simulink model "Model"  (R2021b)
settings: Solver=FixedStepAuto  StartTime=0.0  StopTime=T  FixedStep=0.1  RelTol=1e-3
values from neighbouring files (symbols this model uses):
  A = zeros(length(w_0))    [Model_script.m]
  a = R_E + 550    [Model_script.m]    (also in Orbit_Model.m)
  A0 = eye(3)    [Model_script.m]
  actuators_matrix = [1 0 0; 0 1 0; 0 0 1]    [Model_script.m]
  alpha = deg2rad(11.5)    [Model_script.m]
  Area_mb = diag([A1 A2 A3 A4 A5 A6])    [Model_script.m]
  Area_sp = diag([A7 A8 A9 A10])    [Model_script.m]
  around_boresight = deg2rad(dms2degrees([0,0,around_boresight]))    [Model_script.m]
  B = diag([1/Ix, 1/Iy, 1/Iz])    [Model_script.m]
  cross_boresight = deg2rad(dms2degrees([0,0,cross_boresight]))    [Model_script.m]
  e = 0.0001824    [Model_script.m]    (also in Orbit_Model.m)
  epsilon = deg2rad(23.45)    [Model_script.m]
  H0 = ( g1_0^2 + g1_1^2 + h1_1^2 )^(1/2)    (= 3.0115258674e-05)    [Model_script.m]
  h_N_target = [0; 0; I(3,3)*n]    [Model_script.m]
  I = I_mb + I_depl    [Model_script.m]
  i = deg2rad(53.0545)    [Model_script.m]    (also in Orbit_Model.m)
  I_inv = inv(I)    [Model_script.m]
  i_matrix = [1 0 0; 0 cos(i) sin(i); 0 -sin(i) cos(i)]    [Model_script.m]
  Kb = 1e10    (= 10000000000)    [Model_script.m]
  Kd = 5*1e-4*ones(length(w_0),1)    [Model_script.m]
  Kp = 5*1e-3*ones(length(w_0),1)    [Model_script.m]
  m = [0.01; 0.05; 0.01]    [Model_script.m]
  m_N_unit = zeros(size(m_N,1),size(m_N,2))    [Model_script.m]
  mu_E = astroConstants(13)    [Model_script.m]    (also in Orbit_Model.m)
  n = sqrt(mu_E/(a^3))    [Model_script.m]    (also in Orbit_Model.m)
  n4 = -n1    [Model_script.m]
  N_b_mb = [n1'; n2'; n3'; n4'; n5'; n6']    [Model_script.m]
  N_b_sp = [n7'; n8'; n9'; n10']    [Model_script.m]
  n_sun = 2*pi/T_sun    (= 1.99238499086e-07)    [Model_script.m]
  P = Fe/c    (= 4.52666666667e-06)    [Model_script.m]
  Q = zeros(length(w_0))    [Model_script.m]
  R = zeros(length(w_0))    [Model_script.m]
  R_E = astroConstants(23)    [Model_script.m]    (also in Orbit_Model.m)
  r_mb = [base/2 0 0; 0 base/2 0; 0 0 height/2; -base/2 0 0; 0 -base/2 0; 0 0 -height/2]    [Model_script.m]
  r_sp = [0 length_p1/2+base/2 0; 0 length_p1/2+base/2 0; 0 -length_p2/2-base/2 0; 0 -length_p2/2-base/2 0]    [Model_script.m]
  rho_s_mb = 0.3    [Model_script.m]
  rho_s_sp = 0    [Model_script.m]
  Rs = astroConstants(2)    [Model_script.m]
  star_sensor_tolerance = deg2rad(star_sensor_tolerance)    [Model_script.m]
  theta0 = deg2rad(0)    [Model_script.m]    (also in Orbit_Model.m)
  unit = [1 0 0]'    [Model_script.m]
  v1 = [0 1 -1]'    [Model_script.m]
  v2 = [-1 0 1]'    [Model_script.m]
  v3 = [1 -1 0]'    [Model_script.m]
  w_0 = [wx_0 wy_0 wz_0]'    [Model_script.m]
  w_E = deg2rad(15.04)/3600    [Model_script.m]    (also in Orbit_Model.m = deg2rad(15.04/3600))
  w_target = [0; 0; n]    [Model_script.m]
  weight = 1/6    (= 0.166666666667)    [Model_script.m]
  wy_0 = 0.7    [Model_script.m]
undefined symbols (not defined in the file or in its folder): phi0, psi0, q0
libraries: matrix_library x15, vrlib x12, dspmtrx3 x3, sharedutil x2
(part 1 of 2)
settings Model: Creator=sferl  LastModifiedBy=samuz

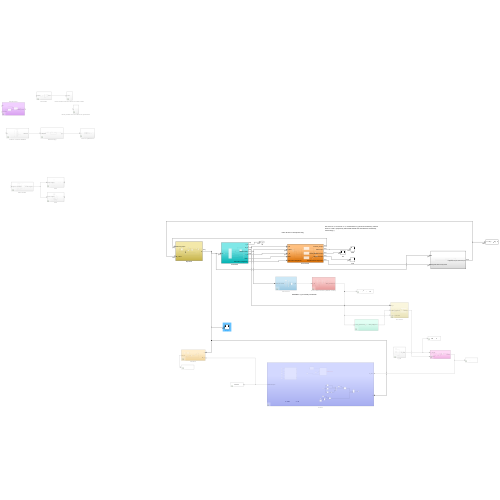
[thumbnail: Simulink's stored preview of the top-level diagram]
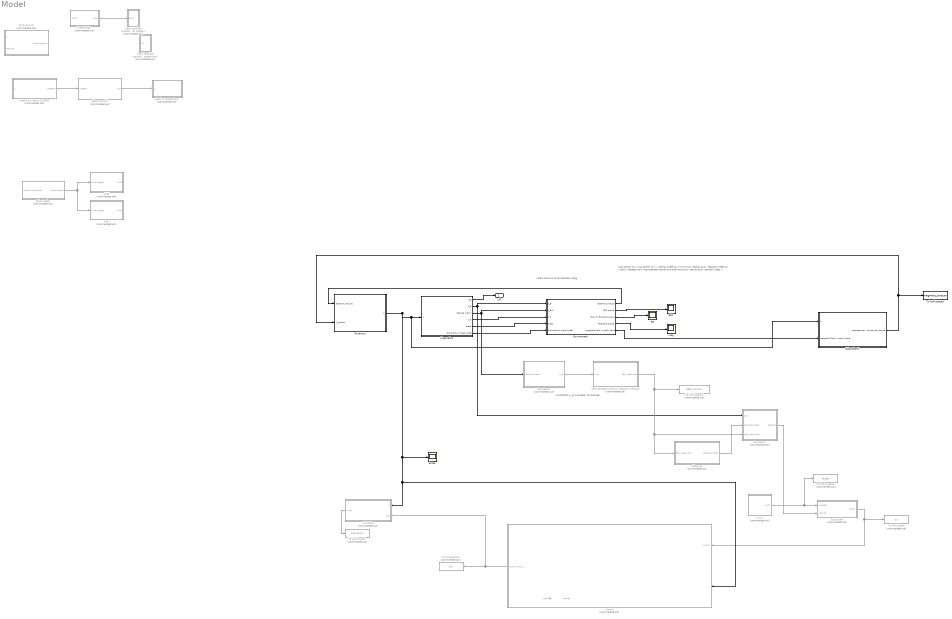
== system Model ==
  note: x = w
  note: u = MC
  note: insert calculus on atmospheric drag
  note: star sensor on z, sun sensor on -x, inertial wheel on y (minimum inertial axis), reaction wheel on x and z (respectively intermediate inertial axis and maximum inertial axis), pannelli lungo y
  note: WARNING: m_B is already normalized!
  A312 : Subsystem  Commented=on
  A313 : Subsystem  Commented=on
  A_L/N : Subsystem  Commented=on
  Actuators : Subsystem  Commented=on
  Attitude Determination (Statistic method) : Subsystem  Commented=on
  Control : Subsystem  Commented=on
  Dynamics : Subsystem
  Environment : Subsystem
  Euler Angles : Subsystem  Commented=on
  GG : Scope
  Kinematics : Subsystem
  Observer : Subsystem  Commented=on
  Pointing error : Subsystem  Commented=on
  SRP : Scope
  Scope : Scope
  Star Sensor : Subsystem  Commented=on
  Subsystem : Subsystem  Commented=on
  Subsystem1 : Subsystem
  Sun sensor : Subsystem  Commented=on
  To Workspace : ToWorkspace  Commented=on  VariableName=err  SampleTime=-1
  To Workspace1 : ToWorkspace  Commented=on  VariableName=actuators  SampleTime=-1
  To Workspace2 : ToWorkspace  Commented=on  VariableName=ctrl  SampleTime=-1
  To Workspace3 : ToWorkspace  Commented=on  VariableName=target  SampleTime=-1
  To Workspace4 : ToWorkspace  Commented=on  VariableName=ABN_sensor  SampleTime=-1
  To Workspace5 : ToWorkspace  VariableName=magnetic_torquer  SampleTime=-1
  check on quaternions : Subsystem  Commented=on
  check possible transformation into euler angles1 : Subsystem  Commented=on
  check possible transformation into quaternions : Subsystem  Commented=on
  creation of matrix \OMEGA : Subsystem  Commented=on
  determne q(t) : Subsystem  Commented=on
  mag : Scope
  trace finder : Subsystem  Commented=on
  r_B : Outport
  wires:
  Kinematics/1(r_B) -> r_B/1
  Kinematics/3(Attitude matrix) -> Environment/2(A_B/N), Star Sensor/1(Attitude matrix)
  Star Sensor/1(m_B) -> Attitude Determination (Statistic method)/1(m_B)
  Kinematics/2(S_B) -> Environment/1(S_B), Sun sensor/1(S_B)
  Kinematics/4(r_N) -> Environment/3(r_N)
  Kinematics/5(theta) -> Environment/4(theta)
  Kinematics/6(Orbit radius (magnitude)) -> Environment/5(Orbit radius (magnitude))
  Environment/1(External_Torque) -> Dynamics/1(External_Torque)
  Attitude Determination (Statistic method)/1(ABN_measured) -> To Workspace4/1, Sun sensor/3(ABN_measured), Observer/1(ABN_measured)
  Observer/1(ABN_estimated) -> Sun sensor/2(ABN_estimated)
  Euler Angles/1(Euler angles) -> A312/1(Euler angles), A313/1(Euler angles)
  Sun sensor/1(Attitude) -> Subsystem/2(Attitude)
  Actuators/1(M_ref) -> To Workspace1/1
  Subsystem/1(error2) -> To Workspace/1, Control/1(A_error)
  creation of matrix \OMEGA/1(\OMEGA) -> determne q(t)/1(OMEGA)
  determne q(t)/1(q(t)) -> check on quaternions/1(q)
  trace finder/1(trace) -> check possible transformation into euler angles1/1(trace)
  Control/1(control torque) -> Actuators/2(M_C), To Workspace2/1
  Environment/2(SRP torque) -> SRP/1
  Environment/3(Gravity Gradient torque) -> GG/1
  Environment/4(Magnetic torque) -> mag/1
  A_L/N/1(A_L/N) -> To Workspace3/1, Subsystem/1(A_target)
  Dynamics/1(w) -> Subsystem1/1(w), Kinematics/1(w), Scope/1, Actuators/1(w), Control/2(w)
  Environment/5(magnetic field in body frame) -> Subsystem1/2(magnetic filed in body frame)
  Subsystem1/1(magnetic torquer control torque) -> To Workspace5/1, Dynamics/2(M_control)

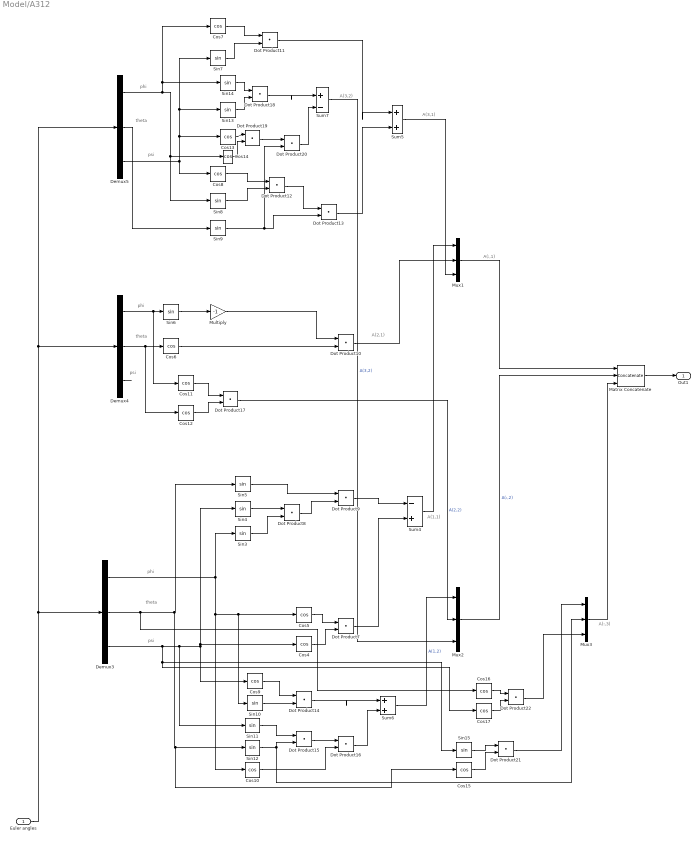
== system Model/A312 ==
  note: A(:,3)
  note: A(3,2)
  note: A(:,1)
  note: A(3,1)
  note: A(2,1)
  note: A(1,1)
  note: psi
  note: psi
  note: theta
  note: phi
  note: phi
  note: theta
  note: psi
  note: phi
  note: theta
  Euler angles : Inport
  Cos{4..17} (14 alike) : Trigonometry  Operator=cos
  Demux3 : Demux  Outputs=3
  Demux4 : Demux  Outputs=3
  Demux5 : Demux  Outputs=3
  Dot Product{7..22} (16 alike) : DotProduct  InputSameDT=on  OutDataTypeStr=Inherit: Inherit via internal rule
  Matrix Concatenate : Concatenate  NumInputs=3  Mode=Multidimensional array  ConcatenateDimension=2
  Multiply : Gain  Gain=-1
  Mux1 : Mux  Inputs=3
  Mux2 : Mux  Inputs=3
  Mux3 : Mux  Inputs=3
  Sin{3..15} (13 alike) : Trigonometry
  Sum4 : Sum  Inputs=-+
  Sum5 : Sum  Inputs=|++
  Sum6 : Sum  Inputs=|++
  Sum7 : Sum  Inputs=|+-
  Out1 : Outport
  wires:
  Cos15/1 -> Dot Product21/2
  Demux4/1 -> Cos11/1, Sin6/1
  Demux3/3 -> Cos17/1, Sin15/1, Sin11/1, Sin4/1, Cos4/1, Cos9/1
  Cos11/1 -> Dot Product17/1
  Sin11/1 -> Dot Product15/1
  Dot Product10/1 -> Mux1/2
  Demux5/3 -> Cos13/1, Sin7/1, Sin13/1, Cos8/1
  Sin7/1 -> Dot Product11/2
  Demux4/2 -> Cos12/1, Cos6/1
  Dot Product12/1 -> Dot Product13/1
  Dot Product7/1 -> Sum4/2
  Dot Product9/1 -> Sum4/1
  Euler angles/1 -> Demux5/1, Demux4/1, Demux3/1
  Sin9/1 -> Dot Product20/2, Dot Product13/2
  Dot Product11/1 -> Sum5/1
  Sin10/1 -> Dot Product14/2
  Sin5/1 -> Dot Product9/1
  Dot Product15/1 -> Dot Product16/1
  Dot Product18/1 -> Sum7/1
  Sum5/1 -> Mux1/3
  Mux2/1 -> Matrix Concatenate/2  "A(:,2)"
  Demux5/1 -> Sin14/1, Cos7/1, Cos14/1, Sin8/1
  Sin3/1 -> Dot Product8/2
  Demux3/2 -> Cos16/1, Cos15/1, Sin12/1, Sin5/1
  Demux3/1 -> Cos10/1, Sin10/1, Cos5/1, Sin3/1
  Cos6/1 -> Dot Product10/2
  Cos7/1 -> Dot Product11/1
  Dot Product13/1 -> Sum5/2
  Sin6/1 -> Multiply/1
  Sin4/1 -> Dot Product8/1
  Dot Product22/1 -> Mux3/3
  Cos8/1 -> Dot Product12/1
  Multiply/1 -> Dot Product10/1
  Dot Product8/1 -> Dot Product9/2
  Demux4/3 -> ?
  Cos5/1 -> Dot Product7/1
  Demux5/2 -> Sin9/1
  Sin15/1 -> Dot Product21/1
  Dot Product14/1 -> Sum6/1
  Cos10/1 -> Dot Product16/2
  Sin14/1 -> Dot Product18/1
  Sin13/1 -> Dot Product18/2
  Sum6/1 -> Mux2/1  "A(1,2)"
  Dot Product20/1 -> Sum7/2
  Sin8/1 -> Dot Product12/2
  Mux1/1 -> Matrix Concatenate/1
  Sum7/1 -> Mux2/3  "A(3,2)"
  Dot Product21/1 -> Mux3/1
  Cos12/1 -> Dot Product17/2
  Cos9/1 -> Dot Product14/1
  Sum4/1 -> Mux1/1
  Dot Product17/1 -> Mux2/2  "A(2,2)"
  Cos13/1 -> Dot Product19/1
  Cos14/1 -> Dot Product19/2
  Dot Product19/1 -> Dot Product20/1
  Cos16/1 -> Dot Product22/1
  Dot Product16/1 -> Sum6/2
  Cos4/1 -> Dot Product7/2
  Cos17/1 -> Dot Product22/2
  Sin12/1 -> Mux3/2, Dot Product15/2
  Mux3/1 -> Matrix Concatenate/3
  Matrix Concatenate/1 -> Out1/1

== system Model/A313 ==
  Euler angles : Inport
  A(:,1) : Subsystem
  A(:,2) : Subsystem
  A(:,3) : Subsystem
  Matrix Concatenate1 : Concatenate  NumInputs=3  Mode=Multidimensional array  ConcatenateDimension=2
  Out1 : Outport
  wires:
  Euler angles/1 -> A(:,3)/1(In1), A(:,2)/1(In1), A(:,1)/1(In1)
  A(:,3)/1(Out1) -> Matrix Concatenate1/3
  A(:,2)/1(Out1) -> Matrix Concatenate1/2
  A(:,1)/1(Out1) -> Matrix Concatenate1/1
  Matrix Concatenate1/1 -> Out1/1

== system Model/A_L//N ==
  Matrix Concatenate : Concatenate  NumInputs=3  Mode=Multidimensional array  ConcatenateDimension=2
  first column of A_L/N : Subsystem
  second column of A_L/N : Subsystem
  third column of A_L/N : Subsystem
  A_L/N : Outport
  wires:
  second column of A_L/N/1(A_L/N (:,2)) -> Matrix Concatenate/2
  Matrix Concatenate/1 -> A_L/N/1
  first column of A_L/N/1(A_L/N (:,1)) -> Matrix Concatenate/1
  third column of A_L/N/1(A_L/N (:,3)) -> Matrix Concatenate/3

== system Model/Actuators ==
  w : Inport
  M_C : Inport  Port=2
  Constant : Constant  Value=actuators_matrix
  Cross Product : matrix_library/Cross Product
      settings: SourceProductBaseCode=SL
  Gain : Gain  Gain=-1
  Gain1 : Gain  Gain=-1
  Integrator : Integrator  InitialCondition=[0; wy_0; 0]
  Matrix Multiply : Product  Multiplication=Matrix(*)
  Matrix Multiply1 : Product  Multiplication=Matrix(*)
  Pseudoinverse : MATLAB Function  TreatAsAtomicUnit=on
  Sum : Sum  Inputs=|++
  M_ref : Outport
  wires:
  Constant/1 -> Matrix Multiply1/1, Pseudoinverse/1(A)
  Pseudoinverse/1(A_pseudoinv) -> Gain/1
  Gain/1 -> Matrix Multiply/1
  M_C/1 -> Sum/1
  w/1 -> Cross Product/1
  Matrix Multiply/1 -> Gain1/1, Integrator/1  "h_r_dot"
  Integrator/1 -> Matrix Multiply1/2  "h_r"
  Matrix Multiply1/1 -> Cross Product/2
  Cross Product/1 -> Sum/2
  Sum/1 -> Matrix Multiply/2
  Gain1/1 -> M_ref/1  "M_r = h_r_dot"

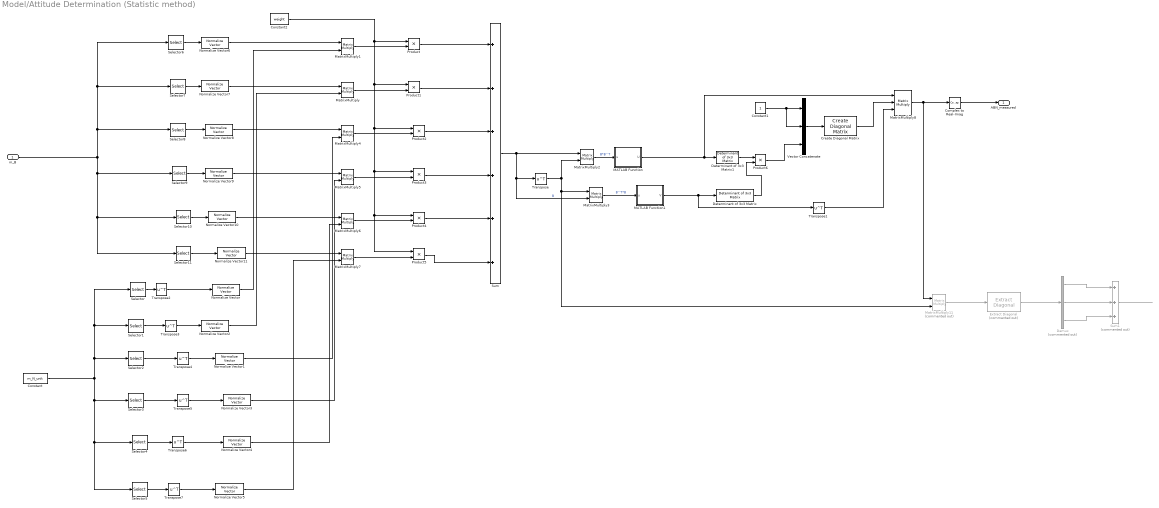
== system Model/Attitude Determination (Statistic method) ==
  m_B : Inport
  Complex to Real-Imag : ComplexToRealImag  Output=Real
  Constant : Constant  Value=m_N_unit
  Constant1 : Constant
  Constant2 : Constant  Value=weight
  Create Diagonal Matrix : dspmtrx3/Create Diagonal Matrix
      settings: SourceProductBaseCode=DS
  Demux : Demux  Commented=on  Outputs=3
  Determinant of 3x3 Matrix : sharedutil/Determinant of 3x3 Matrix  aMode=aMode
      settings: SourceProductBaseCode=AE,PW,DR,MT,UV,VE
  Determinant of 3x3 Matrix1 : sharedutil/Determinant of 3x3 Matrix  aMode=aMode
      settings: SourceProductBaseCode=AE,PW,DR,MT,UV,VE
  Extract Diagonal : dspmtrx3/Extract Diagonal  Commented=on
      settings: SourceProductBaseCode=DS
  MATLAB Function : MATLAB Function  TreatAsAtomicUnit=on
  MATLAB Function1 : MATLAB Function  TreatAsAtomicUnit=on
  MatrixMultiply{,1..7} (8 alike) : Product  Multiplication=Matrix(*)
  MatrixMultiply11 : Product  Commented=on  Multiplication=Matrix(*)
  MatrixMultiply8 : Product  Inputs=3  Multiplication=Matrix(*)
  Normalize Vector{,1..11} (12 alike) : vrlib/Utilities/Normalize Vector  maxzero=0
  Product{,1..6} (7 alike) : Product
  Selector : Selector  NumberOfDimensions=2  InputPortWidth=3  IndexOptions=Starting index (dialog),Starting index (dialog)  Indices=1,1  OutputSizes=3,1
  Selector1 : Selector  NumberOfDimensions=2  InputPortWidth=3  IndexOptions=Starting index (dialog),Starting index (dialog)  Indices=1,2  OutputSizes=3,1
  Selector10 : Selector  NumberOfDimensions=2  InputPortWidth=3  IndexOptions=Starting index (dialog),Starting index (dialog)  Indices=1,5  OutputSizes=3,1
  Selector11 : Selector  NumberOfDimensions=2  InputPortWidth=3  IndexOptions=Starting index (dialog),Starting index (dialog)  Indices=1,6  OutputSizes=3,1
  Selector2 : Selector  NumberOfDimensions=2  InputPortWidth=3  IndexOptions=Starting index (dialog),Starting index (dialog)  Indices=1,3  OutputSizes=3,1
  Selector3 : Selector  NumberOfDimensions=2  InputPortWidth=3  IndexOptions=Starting index (dialog),Starting index (dialog)  Indices=1,4  OutputSizes=3,1
  Selector4 : Selector  NumberOfDimensions=2  InputPortWidth=3  IndexOptions=Starting index (dialog),Starting index (dialog)  Indices=1,5  OutputSizes=3,1
  Selector5 : Selector  NumberOfDimensions=2  InputPortWidth=3  IndexOptions=Starting index (dialog),Starting index (dialog)  Indices=1,6  OutputSizes=3,1
  Selector6 : Selector  NumberOfDimensions=2  InputPortWidth=3  IndexOptions=Starting index (dialog),Starting index (dialog)  Indices=1,1  OutputSizes=3,1
  Selector7 : Selector  NumberOfDimensions=2  InputPortWidth=3  IndexOptions=Starting index (dialog),Starting index (dialog)  Indices=1,2  OutputSizes=3,1
  Selector8 : Selector  NumberOfDimensions=2  InputPortWidth=3  IndexOptions=Starting index (dialog),Starting index (dialog)  Indices=1,3  OutputSizes=3,1
  Selector9 : Selector  NumberOfDimensions=2  InputPortWidth=3  IndexOptions=Starting index (dialog),Starting index (dialog)  Indices=1,4  OutputSizes=3,1
  Sum : Sum  Inputs=++++++
  Sum1 : Sum  Commented=on  Inputs=+++
  Transpose{,1..7} (8 alike) : Math  Operator=transpose  SaturateOnIntegerOverflow=on
  Vector Concatenate : Concatenate  NumInputs=3
  ABN_measured : Outport
  wires:
  Transpose/1 -> MatrixMultiply11/2, MatrixMultiply3/1, MatrixMultiply2/2
  Constant2/1 -> Product3/1, Product4/1, Product5/1, Product2/1, Product1/1, Product/1
  Product2/1 -> Sum/3
  MatrixMultiply/1 -> Product1/2
  Product1/1 -> Sum/2
  MatrixMultiply7/1 -> Product5/2
  Sum/1 -> MatrixMultiply3/2, Transpose/1, MatrixMultiply2/1  "B"
  MatrixMultiply2/1 -> MATLAB Function/1(u)  "B*B^T"
  Product5/1 -> Sum/6
  MatrixMultiply5/1 -> Product3/2
  Product4/1 -> Sum/5
  Product/1 -> Sum/1
  MatrixMultiply4/1 -> Product2/2
  MatrixMultiply1/1 -> Product/2
  Product3/1 -> Sum/4
  MatrixMultiply6/1 -> Product4/2
  Selector1/1 -> Transpose3/1
  Selector3/1 -> Transpose5/1
  Selector4/1 -> Transpose6/1
  Selector2/1 -> Transpose4/1
  Selector5/1 -> Transpose7/1
  m_B/1 -> Selector6/1, Selector7/1, Selector8/1, Selector11/1, Selector10/1, Selector9/1
  Determinant of 3x3 Matrix1/1 -> Product6/1
  Determinant of 3x3 Matrix/1 -> Product6/2
  Constant1/1 -> Vector Concatenate/2, Vector Concatenate/1
  Product6/1 -> Vector Concatenate/3
  Vector Concatenate/1 -> Create Diagonal Matrix/1
  Create Diagonal Matrix/1 -> MatrixMultiply8/2
  MATLAB Function/1(U) -> MatrixMultiply8/1, Determinant of 3x3 Matrix1/1
  Transpose1/1 -> MatrixMultiply8/3
  MatrixMultiply8/1 -> Complex to Real-Imag/1, MatrixMultiply11/1
  MatrixMultiply3/1 -> MATLAB Function1/1(u)  "B^T*B"
  MATLAB Function1/1(V) -> Transpose1/1, Determinant of 3x3 Matrix/1
  MatrixMultiply11/1 -> Extract Diagonal/1
  Extract Diagonal/1 -> Demux/1
  Demux/1 -> Sum1/1
  Demux/2 -> Sum1/2
  Demux/3 -> Sum1/3
  Sum1/1 -> ?
  Selector6/1 -> Normalize Vector6/1
  Selector7/1 -> Normalize Vector7/1
  Selector8/1 -> Normalize Vector8/1
  Selector9/1 -> Normalize Vector9/1
  Selector10/1 -> Normalize Vector10/1
  Selector11/1 -> Normalize Vector11/1
  Selector/1 -> Transpose2/1
  Transpose3/1 -> Normalize Vector2/1
  Transpose2/1 -> Normalize Vector/1
  Transpose4/1 -> Normalize Vector1/1
  Transpose5/1 -> Normalize Vector3/1
  Transpose6/1 -> Normalize Vector4/1
  Transpose7/1 -> Normalize Vector5/1
  Normalize Vector/1 -> MatrixMultiply1/2
  Normalize Vector2/1 -> MatrixMultiply/2
  Normalize Vector1/1 -> MatrixMultiply4/2
  Normalize Vector3/1 -> MatrixMultiply5/2
  Normalize Vector4/1 -> MatrixMultiply6/2
  Normalize Vector5/1 -> MatrixMultiply7/2
  Normalize Vector6/1 -> MatrixMultiply1/1
  Normalize Vector7/1 -> MatrixMultiply/1
  Normalize Vector8/1 -> MatrixMultiply4/1
  Normalize Vector9/1 -> MatrixMultiply5/1
  Normalize Vector10/1 -> MatrixMultiply6/1
  Normalize Vector11/1 -> MatrixMultiply7/1
  Constant/1 -> Selector3/1, Selector4/1, Selector5/1, Selector/1, Selector1/1, Selector2/1
  Complex to Real-Imag/1 -> ABN_measured/1

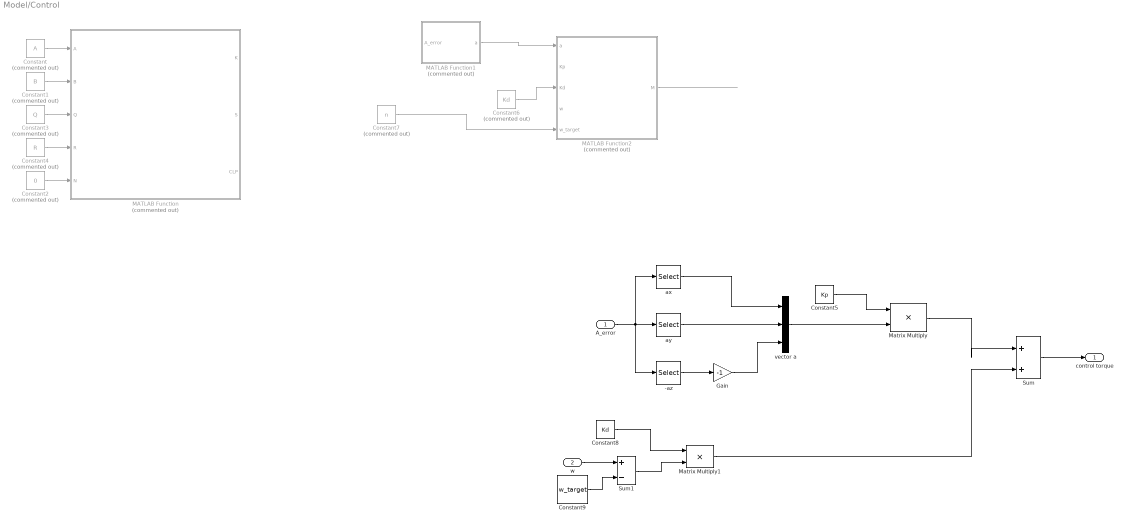
== system Model/Control ==
  A_error : Inport
  w : Inport  Port=2
  -az : Selector  NumberOfDimensions=2  InputPortWidth=3  IndexOptions=Starting index (dialog),Starting index (dialog)  Indices=2,1  OutputSizes=1,1
  Constant : Constant  Commented=on  Value=A
  Constant1 : Constant  Commented=on  Value=B
  Constant2 : Constant  Commented=on  Value=0
  Constant3 : Constant  Commented=on  Value=Q
  Constant4 : Constant  Commented=on  Value=R
  Constant5 : Constant  Value=Kp
  Constant6 : Constant  Commented=on  Value=Kd
  Constant7 : Constant  Commented=on  Value=n
  Constant8 : Constant  Value=Kd
  Constant9 : Constant  Value=w_target
  Gain : Gain  Gain=-1
  MATLAB Function : MATLAB Function  Commented=on  TreatAsAtomicUnit=on
  MATLAB Function1 : MATLAB Function  Commented=on  TreatAsAtomicUnit=on
  MATLAB Function2 : MATLAB Function  Commented=on  TreatAsAtomicUnit=on
  Matrix Multiply : Product
  Matrix Multiply1 : Product
  Sum : Sum  Inputs=|++
  Sum1 : Sum  Inputs=+-
  ax : Selector  NumberOfDimensions=2  InputPortWidth=3  IndexOptions=Starting index (dialog),Starting index (dialog)  Indices=2,3  OutputSizes=1,1
  ay : Selector  NumberOfDimensions=2  InputPortWidth=3  IndexOptions=Starting index (dialog),Starting index (dialog)  Indices=3,1  OutputSizes=1,1
  vector a : Mux  Inputs=3
  control torque : Outport
  wires:
  Constant/1 -> MATLAB Function/1(A)
  Constant1/1 -> MATLAB Function/2(B)
  Constant2/1 -> MATLAB Function/5(N)
  Constant3/1 -> MATLAB Function/3(Q)
  Constant4/1 -> MATLAB Function/4(R)
  MATLAB Function1/1(a) -> MATLAB Function2/1(a)
  Constant6/1 -> MATLAB Function2/3(Kd)
  Constant7/1 -> MATLAB Function2/5(w_target)
  MATLAB Function2/1(M) -> ?
  -az/1 -> Gain/1
  A_error/1 -> ax/1, ay/1, -az/1
  ax/1 -> vector a/1
  ay/1 -> vector a/2
  Gain/1 -> vector a/3
  Constant5/1 -> Matrix Multiply/1
  vector a/1 -> Matrix Multiply/2
  Matrix Multiply/1 -> Sum/1
  Constant8/1 -> Matrix Multiply1/1
  Matrix Multiply1/1 -> Sum/2
  Sum/1 -> control torque/1
  w/1 -> Sum1/1
  Constant9/1 -> Sum1/2
  Sum1/1 -> Matrix Multiply1/2

== system Model/Dynamics ==
  External_Torque : Inport
  M_control : Inport  Port=2
  Constant : Constant  Value=I  VectorParams1D=off
  Constant1 : Constant  Value=I_inv  VectorParams1D=off
  Cross Product : matrix_library/Cross Product
      settings: SourceProductBaseCode=SL
  Integrator : Integrator  InitialCondition=w_0
  Product : Product  Multiplication=Matrix(*)
  Product1 : Product  Multiplication=Matrix(*)
  Sum : Sum  Inputs=|++
  Sum1 : Sum  Inputs=|++
  w : Outport
  wires:
  Product/1 -> Cross Product/1
  Constant/1 -> Product/1
  Constant1/1 -> Product1/1
  Integrator/1 -> Cross Product/2, Product/2, w/1  "w"
  Product1/1 -> Integrator/1  "w_dot"
  Cross Product/1 -> Sum/2
  Sum/1 -> Product1/2
  External_Torque/1 -> Sum1/1
  M_control/1 -> Sum1/2
  Sum1/1 -> Sum/1

== system Model/Environment ==
  S_B : Inport
  A_B/N : Inport  Port=2
  r_N : Inport  Port=3
  theta : Inport  Port=4
  Orbit radius (magnitude) : Inport  Port=5
  GG Torque : Subsystem
  Magnetic Torque : Subsystem
  SRP Torque : Subsystem
  Sum of Torques : Sum  Inputs=+|+|+  CollapseMode=Specified dimension
  To Workspace2 : ToWorkspace  VariableName=mag  SampleTime=-1
  External_Torque : Outport
  SRP torque : Outport  Port=2
  Gravity Gradient torque : Outport  Port=3
  Magnetic torque : Outport  Port=4
  magnetic field in body frame : Outport  Port=5
  wires:
  SRP Torque/1(T_SRP) -> SRP torque/1, Sum of Torques/1
  r_N/1 -> Magnetic Torque/2(r_N)
  GG Torque/1(T_GG) -> Gravity Gradient torque/1, Sum of Torques/2
  A_B/N/1 -> Magnetic Torque/1(A_B/N), GG Torque/1(A_B/N)
  Orbit radius (magnitude)/1 -> GG Torque/3(R_orbit)
  Magnetic Torque/1(T_MAG) -> Magnetic torque/1, To Workspace2/1, Sum of Torques/3
  Sum of Torques/1 -> External_Torque/1
  S_B/1 -> SRP Torque/1(S_B)
  theta/1 -> GG Torque/2(theta)
  Magnetic Torque/2(magnetic field in body frame) -> magnetic field in body frame/1

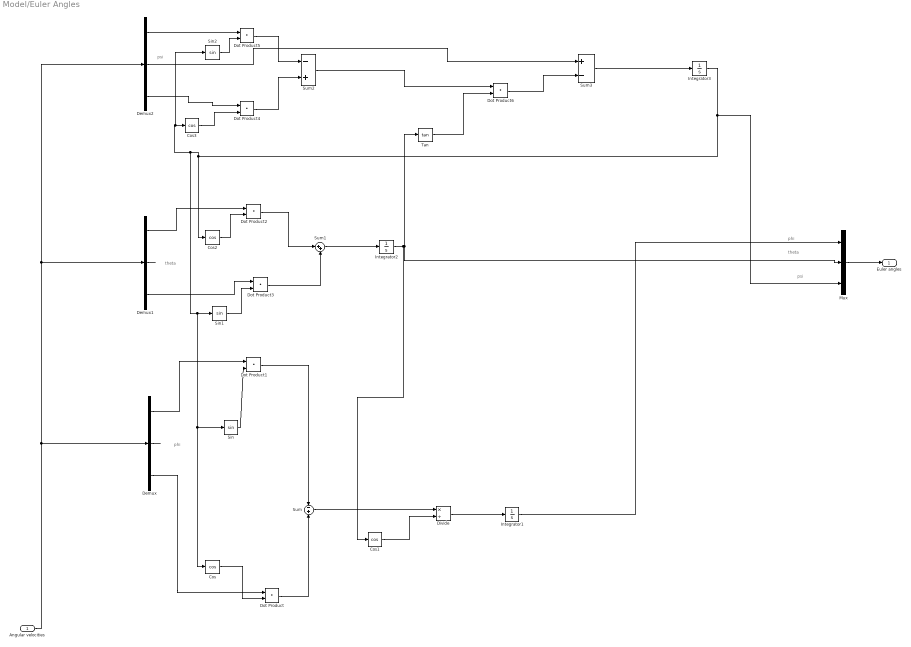
== system Model/Euler Angles ==
  note: psi
  note: theta
  note: phi
  note: psi
  note: theta
  note: phi
  Angular velocities : Inport
  Cos{,1..3} (4 alike) : Trigonometry  Operator=cos
  Demux : Demux  Outputs=3
  Demux1 : Demux  Outputs=3
  Demux2 : Demux  Outputs=3
  Divide : Product  Inputs=*/
  Dot Product{,1..6} (7 alike) : DotProduct  InputSameDT=on  OutDataTypeStr=Inherit: Inherit via internal rule
  Integrator1 : Integrator  InitialCondition=phi0
  Integrator2 : Integrator  InitialCondition=theta0
  Integrator3 : Integrator  InitialCondition=psi0
  Mux : Mux  Inputs=3
  Sin : Trigonometry
  Sin1 : Trigonometry
  Sin2 : Trigonometry
  Sum : Sum  Inputs=-+
  Sum1 : Sum  Inputs=|++
  Sum2 : Sum  Inputs=-+
  Sum3 : Sum  Inputs=+-
  Tan : Trigonometry  Operator=tan
  Euler angles : Outport
  wires:
  Demux/1 -> Dot Product1/1
  Dot Product3/1 -> Sum1/2
  Sum/1 -> Divide/1
  Cos/1 -> Dot Product/2
  Dot Product1/1 -> Sum/1
  Integrator1/1 -> Mux/1
  Sum1/1 -> Integrator2/1
  Integrator2/1 -> Mux/2, Tan/1, Cos1/1
  Dot Product/1 -> Sum/2
  Demux1/3 -> Dot Product3/1
  Angular velocities/1 -> Demux2/1, Demux1/1, Demux/1
  Divide/1 -> Integrator1/1
  Dot Product6/1 -> Sum3/2
  Demux2/1 -> Dot Product5/1
  Sum2/1 -> Dot Product6/1
  Dot Product4/1 -> Sum2/2
  Dot Product2/1 -> Sum1/1
  Demux1/2 -> ?
  Sin/1 -> Dot Product1/2
  Tan/1 -> Dot Product6/2
  Sin1/1 -> Dot Product3/2
  Demux2/3 -> Dot Product4/1
  Cos2/1 -> Dot Product2/2
  Demux2/2 -> Sum3/1
  Cos3/1 -> Dot Product4/2
  Cos1/1 -> Divide/2
  Integrator3/1 -> Cos/1, Sin/1, Sin1/1, Sin2/1, Cos3/1, Cos2/1, Mux/3
  Dot Product5/1 -> Sum2/1
  Demux/3 -> Dot Product/1
  Sin2/1 -> Dot Product5/2
  Sum3/1 -> Integrator3/1
  Demux1/1 -> Dot Product2/1
  Demux/2 -> ?
  Mux/1 -> Euler angles/1

== system Model/Kinematics ==
  w : Inport
  Sun direction with respect to body frame (already normalized!) : Subsystem
  "radius of orbit in body frame and transformation matrix from inertial frame to body frame " : Subsystem
  r_B : Outport
  S_B : Outport  Port=2
  Attitude matrix : Outport  Port=3
  r_N : Outport  Port=4
  theta : Outport  Port=5
  Orbit radius (magnitude) : Outport  Port=6
  wires:
  "radius of orbit in body frame and transformation matrix from inertial frame to body frame "/1(r_B) -> r_B/1
  w/1 -> "radius of orbit in body frame and transformation matrix from inertial frame to body frame "/1(w)
  Sun direction with respect to body frame (already normalized!)/1(S_B) -> S_B/1
  "radius of orbit in body frame and transformation matrix from inertial frame to body frame "/3(r_N) -> r_N/1
  "radius of orbit in body frame and transformation matrix from inertial frame to body frame "/4(theta) -> theta/1
  "radius of orbit in body frame and transformation matrix from inertial frame to body frame "/5(R_orbit) -> Orbit radius (magnitude)/1
  "radius of orbit in body frame and transformation matrix from inertial frame to body frame "/2(A_B/N) -> Attitude matrix/1, Sun direction with respect to body frame (already normalized!)/1(A_B/N)

== system Model/Observer ==
  ABN_measured : Inport
  Gain : Gain  Gain=0.5
  ABN_estimated : Outport
  wires:
  ABN_measured/1 -> Gain/1
  Gain/1 -> ABN_estimated/1

== system Model/Pointing error ==
  w : Inport
  Attitude : Inport  Port=2
  Angular momentum in body frame : Subsystem
  pointing error evaluated in inertial frame : Subsystem
  pointing error : Outport
  wires:
  w/1 -> Angular momentum in body frame/1(w)
  Angular momentum in body frame/1(h_B) -> pointing error evaluated in inertial frame/2(h_B)
  Attitude/1 -> pointing error evaluated in inertial frame/1(A_B/N)
  pointing error evaluated in inertial frame/1(err) -> pointing error/1

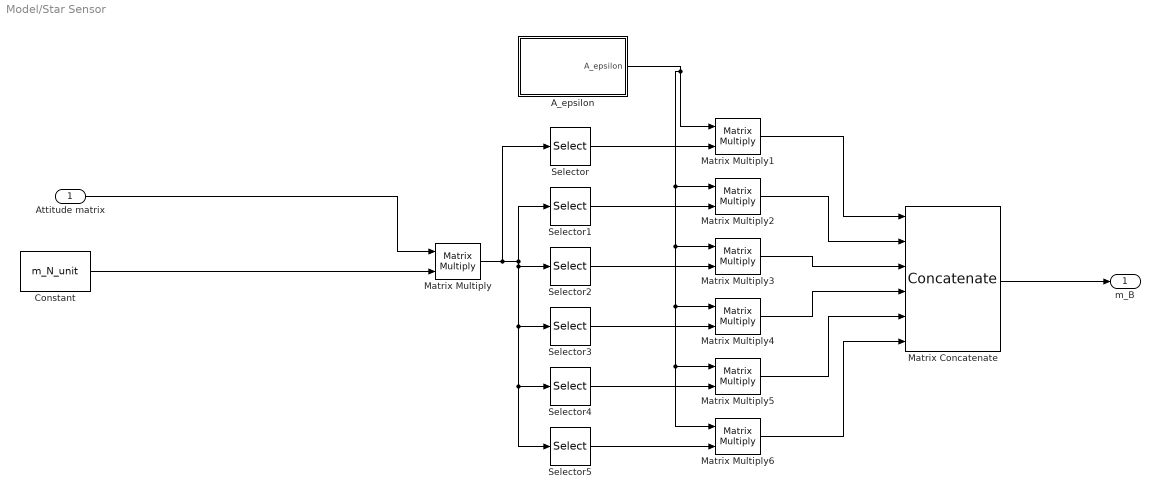
== system Model/Star Sensor ==
  Attitude matrix : Inport
  A_epsilon : Subsystem
  Constant : Constant  Value=m_N_unit
  Matrix Concatenate : Concatenate  NumInputs=6  Mode=Multidimensional array  ConcatenateDimension=2
  Matrix Multiply{,1..6} (7 alike) : Product  Multiplication=Matrix(*)
  Selector : Selector  NumberOfDimensions=2  InputPortWidth=3  IndexOptions=Starting index (dialog),Starting index (dialog)  Indices=1,1  OutputSizes=3,1
  Selector1 : Selector  NumberOfDimensions=2  InputPortWidth=3  IndexOptions=Starting index (dialog),Starting index (dialog)  Indices=1,2  OutputSizes=3,1
  Selector2 : Selector  NumberOfDimensions=2  InputPortWidth=3  IndexOptions=Starting index (dialog),Starting index (dialog)  Indices=1,3  OutputSizes=3,1
  Selector3 : Selector  NumberOfDimensions=2  InputPortWidth=3  IndexOptions=Starting index (dialog),Starting index (dialog)  Indices=1,4  OutputSizes=3,1
  Selector4 : Selector  NumberOfDimensions=2  InputPortWidth=3  IndexOptions=Starting index (dialog),Starting index (dialog)  Indices=1,5  OutputSizes=3,1
  Selector5 : Selector  NumberOfDimensions=2  InputPortWidth=3  IndexOptions=Starting index (dialog),Starting index (dialog)  Indices=1,6  OutputSizes=3,1
  m_B : Outport
  wires:
  Attitude matrix/1 -> Matrix Multiply/1
  Constant/1 -> Matrix Multiply/2
  Matrix Multiply/1 -> Selector5/1, Selector4/1, Selector3/1, Selector2/1, Selector1/1, Selector/1
  A_epsilon/1(A_epsilon) -> Matrix Multiply6/1, Matrix Multiply5/1, Matrix Multiply4/1, Matrix Multiply3/1, Matrix Multiply2/1, Matrix Multiply1/1
  Selector/1 -> Matrix Multiply1/2
  Selector1/1 -> Matrix Multiply2/2
  Selector2/1 -> Matrix Multiply3/2
  Selector3/1 -> Matrix Multiply4/2
  Selector4/1 -> Matrix Multiply5/2
  Selector5/1 -> Matrix Multiply6/2
  Matrix Multiply1/1 -> Matrix Concatenate/1
  Matrix Multiply2/1 -> Matrix Concatenate/2
  Matrix Multiply3/1 -> Matrix Concatenate/3
  Matrix Multiply4/1 -> Matrix Concatenate/4
  Matrix Multiply5/1 -> Matrix Concatenate/5
  Matrix Multiply6/1 -> Matrix Concatenate/6
  Matrix Concatenate/1 -> m_B/1

== system Model/Subsystem ==
  note: A measured
  note: A target
  A_target : Inport
  Attitude : Inport  Port=2
  Matrix Multiply : Product  Multiplication=Matrix(*)
  Transpose : Math  Operator=transpose  SaturateOnIntegerOverflow=on
  error2 : Outport
  wires:
  Transpose/1 -> Matrix Multiply/2
  Matrix Multiply/1 -> error2/1
  Attitude/1 -> Matrix Multiply/1
  A_target/1 -> Transpose/1

== system Model/Subsystem1 ==
  note: B_dot
  w : Inport
  magnetic filed in body frame : Inport  Port=2
  Constant : Constant  Value=Kb
  Cross Product : matrix_library/Cross Product
      settings: SourceProductBaseCode=SL
  Demux : Demux  Outputs=3
  Gain : Gain  Gain=-1
  Gain1 : Gain  Gain=-1
  Matrix Multiply : Product  Multiplication=Matrix(*)
  Matrix Multiply1 : Product
  w_hat : Subsystem
  magnetic torquer control torque : Outport
  wires:
  Matrix Multiply/1 -> Matrix Multiply1/2
  Demux/3 -> w_hat/3(w_z)  "w_z"
  magnetic filed in body frame/1 -> Cross Product/2, Matrix Multiply/2
  Gain/1 -> Matrix Multiply1/1
  Gain1/1 -> Matrix Multiply/1
  Demux/1 -> w_hat/1(w_x)  "w_x"
  Cross Product/1 -> magnetic torquer control torque/1
  w_hat/1(w_hat) -> Gain1/1
  Demux/2 -> w_hat/2(w_y)  "w_y"
  Matrix Multiply1/1 -> Cross Product/1
  Constant/1 -> Gain/1
  w/1 -> Demux/1

== system Model/Sun sensor ==
  note: If cos(angle) is negative then the star sensor is not pointing towards the Sun -> star sensor is turned on and I compute the attitude with its measurements (see attitude determination block)
  note: if cos(angle) is positive then the star sensor is pointing towards the Sun -> star sensor must be turned off and I activate the observer to estimate the attitude from the latest given measurements
  S_B : Inport
  ABN_estimated : Inport  Port=2
  ABN_measured : Inport  Port=3
  Constant : Constant  Value=n4
  Constant3 : Constant  Value=star_sensor_tolerance
  Cos : Trigonometry  Operator=cos
  Dot Product : DotProduct  InputSameDT=on  OutDataTypeStr=Inherit: Inherit via internal rule
  Sum : Sum  Inputs=+-
  Switch : Switch  Criteria=u2 > Threshold
  Attitude : Outport
  wires:
  S_B/1 -> Dot Product/1
  Dot Product/1 -> Sum/1  "cos(angle_between_n3_and_Sb)"
  ABN_estimated/1 -> Switch/1  "star sensor points Sun"
  ABN_measured/1 -> Switch/3  "star sensor doesn't point Sun"
  Switch/1 -> Attitude/1
  Constant3/1 -> Cos/1
  Cos/1 -> Sum/2
  Sum/1 -> Switch/2
  Constant/1 -> Dot Product/2

== system Model/check on quaternions ==
  q : Inport
  Demux4 : Demux
  Dot Product{,1..3} (4 alike) : DotProduct  InputSameDT=on  OutDataTypeStr=Inherit: Inherit via internal rule
  Sum : Sum  Inputs=|++++
  To Workspace3 : ToWorkspace  VariableName=check  SampleTime=-1
  wires:
  Demux4/2 -> Dot Product1/1, Dot Product1/2
  Demux4/4 -> Dot Product3/1, Dot Product3/2
  Dot Product3/1 -> Sum/4
  Dot Product1/1 -> Sum/2
  Demux4/3 -> Dot Product2/1, Dot Product2/2
  Dot Product/1 -> Sum/1
  Demux4/1 -> Dot Product/1, Dot Product/2
  Dot Product2/1 -> Sum/3
  Sum/1 -> To Workspace3/1
  q/1 -> Demux4/1

== system Model/check possible transformation into euler angles1 ==
  trace : Inport
  Acos : Trigonometry  Operator=acos
  Constant : Constant
  Gain : Gain  Gain=0.5
  Scope : Scope
  Sin : Trigonometry
  Sum : Sum  Inputs=+-
  wires:
  Sin/1 -> Scope/1
  Sum/1 -> Gain/1
  Constant/1 -> Sum/2
  Acos/1 -> Sin/1
  Gain/1 -> Acos/1
  trace/1 -> Sum/1

== system Model/check possible transformation into quaternions ==
  In1 : Inport
  Acos : Trigonometry  Operator=acos
  Constant : Constant
  Gain : Gain  Gain=0.5
  Scope : Scope
  Sin : Trigonometry
  Sum : Sum  Inputs=+-
  wires:
  Sin/1 -> Scope/1
  Sum/1 -> Gain/1
  Constant/1 -> Sum/2
  Acos/1 -> Sin/1
  Gain/1 -> Acos/1
  In1/1 -> Sum/1

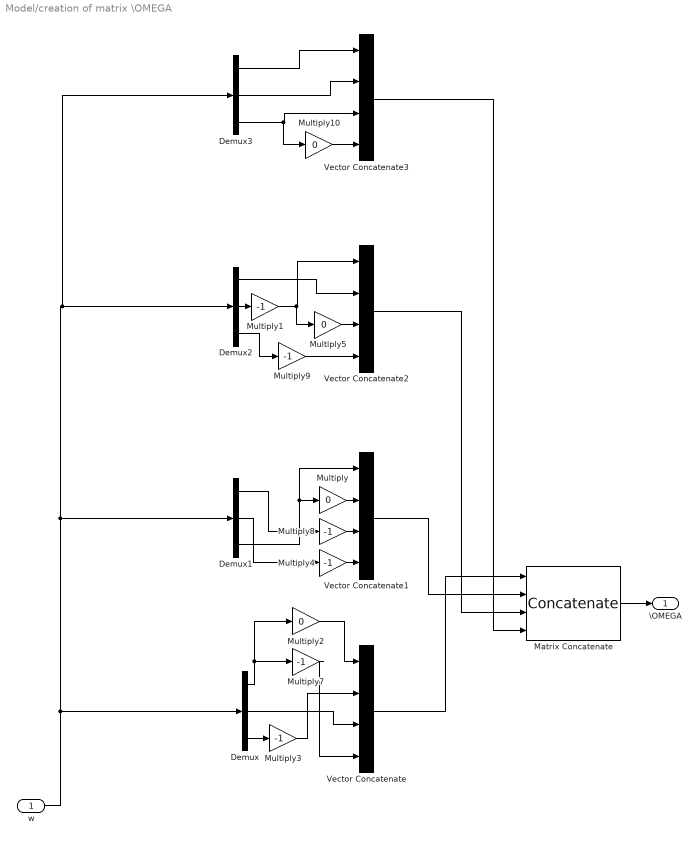
== system Model/creation of matrix \OMEGA ==
  w : Inport
  Demux{,1..3} (4 alike) : Demux  Outputs=3
  Matrix Concatenate : Concatenate  NumInputs=4  Mode=Multidimensional array  ConcatenateDimension=2
  Multiply{,2,5,10} (4 alike) : Gain  Gain=0
  Multiply{1,3..4,7..9} (6 alike) : Gain  Gain=-1
  Vector Concatenate{,1..3} (4 alike) : Concatenate  NumInputs=4
  \OMEGA : Outport
  wires:
  Multiply7/1 -> Vector Concatenate/4
  Vector Concatenate/1 -> Matrix Concatenate/1
  Multiply2/1 -> Vector Concatenate/1
  Vector Concatenate3/1 -> Matrix Concatenate/4
  Demux1/1 -> Multiply8/1
  Multiply9/1 -> Vector Concatenate2/4
  Demux2/2 -> Multiply1/1
  Multiply1/1 -> Multiply5/1, Vector Concatenate2/1
  Demux/1 -> Multiply2/1, Multiply7/1
  Demux3/1 -> Vector Concatenate3/1
  w/1 -> Demux3/1, Demux2/1, Demux1/1, Demux/1
  Demux1/3 -> Multiply/1, Vector Concatenate1/1
  Vector Concatenate1/1 -> Matrix Concatenate/2
  Multiply8/1 -> Vector Concatenate1/3
  Demux/3 -> Multiply3/1
  Vector Concatenate2/1 -> Matrix Concatenate/3
  Matrix Concatenate/1 -> \OMEGA/1
  Multiply/1 -> Vector Concatenate1/2
  Multiply5/1 -> Vector Concatenate2/3
  Demux1/2 -> Multiply4/1
  Demux/2 -> Vector Concatenate/3
  Demux2/3 -> Multiply9/1
  Multiply4/1 -> Vector Concatenate1/4
  Multiply10/1 -> Vector Concatenate3/4
  Demux3/2 -> Vector Concatenate3/2
  Multiply3/1 -> Vector Concatenate/2
  Demux3/3 -> Multiply10/1, Vector Concatenate3/3
  Demux2/1 -> Vector Concatenate2/2

== system Model/determne q(t) ==
  OMEGA : Inport
  Integrator1 : Integrator  InitialCondition=q0
  Matrix Multiply1 : Product  Multiplication=Matrix(*)
  Multiply11 : Gain  Gain=1/2
  q(t) : Outport
  wires:
  OMEGA/1 -> Multiply11/1
  Matrix Multiply1/1 -> Integrator1/1
  Integrator1/1 -> q(t)/1, Matrix Multiply1/2
  Multiply11/1 -> Matrix Multiply1/1

== system Model/trace finder ==
  matrix : Inport
  Demux : Demux  Outputs=3
  Extract Diagonal : dspmtrx3/Extract Diagonal
      settings: SourceProductBaseCode=DS
  Sum1 : Sum  Inputs=+++
  trace : Outport
  wires:
  Sum1/1 -> trace/1
  Demux/1 -> Sum1/1
  Demux/2 -> Sum1/2
  Extract Diagonal/1 -> Demux/1
  Demux/3 -> Sum1/3
  matrix/1 -> Extract Diagonal/1

== system Model/A313/A(:,1) ==
  In1 : Inport
  Demux6 : Demux  Outputs=3
  Subsystem : Subsystem
  Subsystem1 : Subsystem
  Subsystem2 : Subsystem
  Vector Concatenate : Concatenate  NumInputs=3
  Out1 : Outport
  wires:
  Subsystem2/1(A(3,1)) -> Vector Concatenate/3
  Demux6/1 -> Subsystem2/1(phi), Subsystem1/1(phi), Subsystem/1(phi)  "phi"
  Demux6/3 -> Subsystem1/3(psi), Subsystem/3(psi)  "psi"
  Subsystem1/1(A(2,1)) -> Vector Concatenate/2
  Demux6/2 -> Subsystem2/2(theta), Subsystem1/2(theta), Subsystem/2(theta)  "theta"
  In1/1 -> Demux6/1
  Subsystem/1(A(1,1)) -> Vector Concatenate/1
  Vector Concatenate/1 -> Out1/1

== system Model/A313/A(:,2) ==
  In1 : Inport
  Demux7 : Demux  Outputs=3
  Subsystem3 : Subsystem
  Subsystem4 : Subsystem
  Subsystem5 : Subsystem
  Vector Concatenate1 : Concatenate  NumInputs=3
  Out1 : Outport
  wires:
  Demux7/3 -> Subsystem4/3(psi), Subsystem3/3(psi)  "psi"
  Subsystem5/1(A(3,2)) -> Vector Concatenate1/3
  In1/1 -> Demux7/1
  Subsystem4/1(A(2,2)) -> Vector Concatenate1/2
  Demux7/1 -> Subsystem3/1(phi), Subsystem5/1(phi), Subsystem4/1(phi)  "phi"
  Vector Concatenate1/1 -> Out1/1
  Demux7/2 -> Subsystem4/2(theta), Subsystem5/2(theta), Subsystem3/2(theta)  "theta"
  Subsystem3/1(A(1,2)) -> Vector Concatenate1/1

== system Model/A313/A(:,3) ==
  In1 : Inport
  Demux8 : Demux  Outputs=3
  Subsystem6 : Subsystem
  Subsystem7 : Subsystem
  Subsystem8 : Subsystem
  Vector Concatenate2 : Concatenate  NumInputs=3
  Out1 : Outport
  wires:
  Demux8/2 -> Subsystem8/1(theta), Subsystem6/1(theta), Subsystem7/1(theta)  "theta"
  Subsystem7/1(A(2,3)) -> Vector Concatenate2/2
  Vector Concatenate2/1 -> Out1/1
  Subsystem8/1(A(3,3)) -> Vector Concatenate2/3
  Subsystem6/1(A(1,3)) -> Vector Concatenate2/1
  In1/1 -> Demux8/1
  Demux8/3 -> Subsystem7/2(psi), Subsystem6/2(psi)  "psi"

== system Model/A_L//N/first column of A_L//N ==
  Constant : Constant  Value=0
  Cos : Trigonometry  Operator=cos
  Gain : Gain  Gain=-1
  Sin : Trigonometry
  Vector Concatenate : Concatenate  NumInputs=3
  argument of periodic functions : Subsystem
  argument of periodic functions1 : Subsystem
  A_L/N (:,1) : Outport
  wires:
  argument of periodic functions/1(n*t) -> Cos/1
  Constant/1 -> Vector Concatenate/3
  Cos/1 -> Vector Concatenate/1
  Vector Concatenate/1 -> A_L/N (:,1)/1
  Gain/1 -> Vector Concatenate/2
  Sin/1 -> Gain/1
  argument of periodic functions1/1(n*t) -> Sin/1

== system Model/A_L//N/second column of A_L//N ==
  Constant : Constant  Value=0
  Cos : Trigonometry
  Sin : Trigonometry  Operator=cos
  Vector Concatenate : Concatenate  NumInputs=3
  argument of periodic functions : Subsystem
  argument of periodic functions1 : Subsystem
  A_L/N (:,2) : Outport
  wires:
  argument of periodic functions/1(n*t) -> Cos/1
  Constant/1 -> Vector Concatenate/3
  Cos/1 -> Vector Concatenate/1
  Vector Concatenate/1 -> A_L/N (:,2)/1
  Sin/1 -> Vector Concatenate/2
  argument of periodic functions1/1(n*t) -> Sin/1

== system Model/A_L//N/third column of A_L//N ==
  Constant : Constant
  Constant1 : Constant  Value=0
  Constant2 : Constant  Value=0
  Vector Concatenate : Concatenate  NumInputs=3
  A_L/N (:,3) : Outport
  wires:
  Constant/1 -> Vector Concatenate/3
  Vector Concatenate/1 -> A_L/N (:,3)/1
  Constant1/1 -> Vector Concatenate/2
  Constant2/1 -> Vector Concatenate/1

== system Model/Environment/GG Torque ==
  A_B/N : Inport
  theta : Inport  Port=2
  R_orbit : Inport  Port=3
  Gravity Gradient : Subsystem
  Transformation from A_B/N to A_B/L : Subsystem
  T_GG : Outport
  wires:
  Gravity Gradient/1(T_GG) -> T_GG/1
  Transformation from A_B/N to A_B/L/1(A_B/L) -> Gravity Gradient/1(A_BL)
  A_B/N/1 -> Transformation from A_B/N to A_B/L/1(A_B/N)
  theta/1 -> Transformation from A_B/N to A_B/L/2(theta)
  R_orbit/1 -> Gravity Gradient/2(R_orbit)

== system Model/Environment/Magnetic Torque ==
  A_B/N : Inport
  r_N : Inport  Port=2
  Cross Product : matrix_library/Cross Product
      settings: SourceProductBaseCode=SL
  magnetic field of Earth (modelled as dipole) in body frame : Subsystem
  parasitic magnetic torque : Constant  Value=m
  T_MAG : Outport
  magnetic field in body frame : Outport  Port=2
  wires:
  A_B/N/1 -> magnetic field of Earth (modelled as dipole) in body frame/1(A_B/N)
  magnetic field of Earth (modelled as dipole) in body frame/1(b_B) -> magnetic field in body frame/1, Cross Product/2
  parasitic magnetic torque/1 -> Cross Product/1
  Cross Product/1 -> T_MAG/1
  r_N/1 -> magnetic field of Earth (modelled as dipole) in body frame/2(r_N)

== system Model/Environment/SRP Torque ==
  S_B : Inport
  Matrix Concatenate : Concatenate  Mode=Multidimensional array
  SRP Force on spacecraft main body : Subsystem
  SRP Force on spacecraft solar panels : Subsystem
  SRP Torque on spacecraft main body : Subsystem
  SRP Torque on spacecraft solar panels : Subsystem
  Sum of Elements : Sum  Inputs=+  CollapseMode=Specified dimension
  Transpose : Math  Operator=transpose  SaturateOnIntegerOverflow=on
  T_SRP : Outport
  wires:
  S_B/1 -> SRP Force on spacecraft main body/1(S_B), SRP Force on spacecraft solar panels/1(S_B)
  SRP Force on spacecraft solar panels/1(F_sp) -> SRP Torque on spacecraft solar panels/1(F_sp)
  SRP Force on spacecraft main body/1(F_mb) -> SRP Torque on spacecraft main body/1(F_mb)
  SRP Torque on spacecraft solar panels/1(T_sp) -> Matrix Concatenate/2
  SRP Torque on spacecraft main body/1(T_mb) -> Matrix Concatenate/1
  Sum of Elements/1 -> Transpose/1
  Transpose/1 -> T_SRP/1
  Matrix Concatenate/1 -> Sum of Elements/1

== system Model/Kinematics/Sun direction with respect to body frame (already normalized!) ==
  note: I divide the vector for its magnitude (Rs): this is the normalization!
  A_B/N : Inport
  Constant7 : Constant  Value=1/Rs
  MatrixMultiply : Product  Multiplication=Matrix(*)
  Product5 : Product
  S_N : Subsystem
  S_B : Outport
  wires:
  S_N/1(Out1) -> MatrixMultiply/2
  A_B/N/1 -> MatrixMultiply/1
  Constant7/1 -> Product5/1
  MatrixMultiply/1 -> Product5/2
  Product5/1 -> S_B/1

== system Model/Kinematics/radius of orbit in body frame and transformation matrix from inertial frame to body frame  ==
  w : Inport
  MatrixMultiply1 : Product  Multiplication=Matrix(*)
  finder of A_B/N(t) : Subsystem
  orthonormalization of matrix A(t) : Subsystem
  radius of orbit in the inertial reference frame : Subsystem
  r_B : Outport
  A_B/N : Outport  Port=2
  r_N : Outport  Port=3
  theta : Outport  Port=4
  R_orbit : Outport  Port=5
  wires:
  finder of A_B/N(t)/1(A(t)) -> orthonormalization of matrix A(t)/1(A(t))
  orthonormalization of matrix A(t)/1(A_orthonorm) -> A_B/N/1, MatrixMultiply1/2
  MatrixMultiply1/1 -> r_B/1
  radius of orbit in the inertial reference frame/2(r_N) -> MatrixMultiply1/1, r_N/1
  w/1 -> finder of A_B/N(t)/1(w)
  radius of orbit in the inertial reference frame/1(theta) -> theta/1
  radius of orbit in the inertial reference frame/3(R_orbit) -> R_orbit/1

== system Model/Pointing error/Angular momentum in body frame ==
  w : Inport
  Constant1 : Constant  Value=I
  Matrix Multiply : Product  Multiplication=Matrix(*)
  h_B : Outport
  wires:
  w/1 -> Matrix Multiply/2
  Matrix Multiply/1 -> h_B/1
  Constant1/1 -> Matrix Multiply/1

== system Model/Pointing error/pointing error evaluated in inertial frame ==
  A_B/N : Inport
  h_B : Inport  Port=2
  Pointing error : Subsystem
  angular momentum in inertial frame : Subsystem
  err : Outport
  wires:
  angular momentum in inertial frame/1(h_N) -> Pointing error/1(h_N)
  Pointing error/1(err) -> err/1
  A_B/N/1 -> angular momentum in inertial frame/1(A_B/N)
  h_B/1 -> angular momentum in inertial frame/2(h_B)

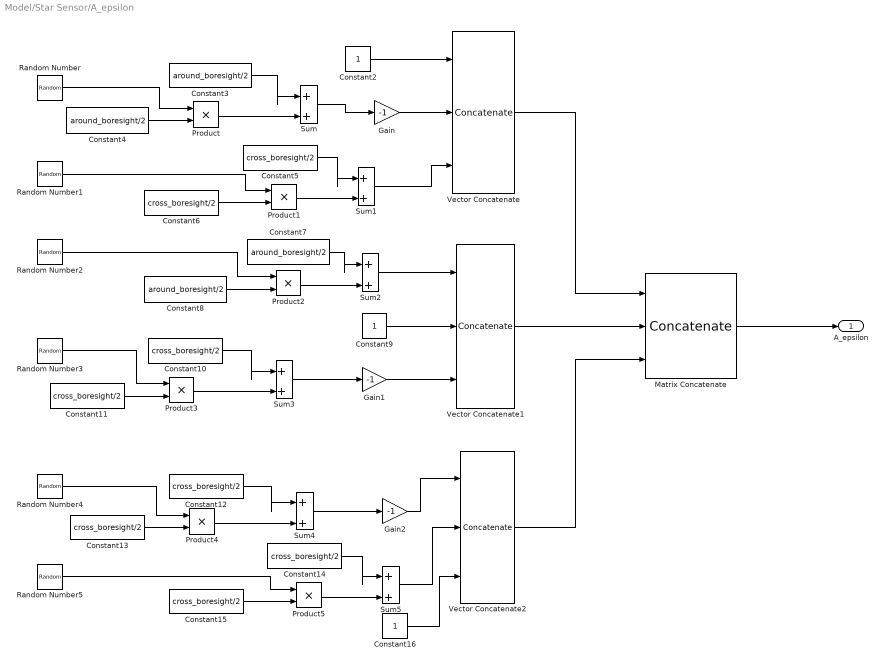
== system Model/Star Sensor/A_epsilon ==
  Constant{5..6,10..15} (8 alike) : Constant  Value=cross_boresight/2
  Constant16 : Constant
  Constant2 : Constant
  Constant{3..4,7..8} (4 alike) : Constant  Value=around_boresight/2
  Constant9 : Constant
  Gain : Gain  Gain=-1
  Gain1 : Gain  Gain=-1
  Gain2 : Gain  Gain=-1
  Matrix Concatenate : Concatenate  NumInputs=3  Mode=Multidimensional array  ConcatenateDimension=2
  Product{,1..5} (6 alike) : Product
  Random Number{,1..5} (6 alike) : RandomNumber  Variance=0.16  SampleTime=0.1
  Sum{,1..5} (6 alike) : Sum  Inputs=|++
  Vector Concatenate : Concatenate  NumInputs=3  Mode=Multidimensional array
  Vector Concatenate1 : Concatenate  NumInputs=3  Mode=Multidimensional array
  Vector Concatenate2 : Concatenate  NumInputs=3  Mode=Multidimensional array
  A_epsilon : Outport
  wires:
  Constant10/1 -> Sum3/1
  Random Number/1 -> Product/1
  Constant12/1 -> Sum4/1
  Vector Concatenate2/1 -> Matrix Concatenate/3
  Constant11/1 -> Product3/2
  Sum/1 -> Gain/1
  Vector Concatenate1/1 -> Matrix Concatenate/2
  Constant3/1 -> Sum/1
  Product1/1 -> Sum1/2
  Constant15/1 -> Product5/2
  Constant16/1 -> Vector Concatenate2/3
  Product5/1 -> Sum5/2
  Constant13/1 -> Product4/2
  Product3/1 -> Sum3/2
  Constant6/1 -> Product1/2
  Product2/1 -> Sum2/2
  Constant7/1 -> Sum2/1
  Constant4/1 -> Product/2
  Constant9/1 -> Vector Concatenate1/2
  Constant8/1 -> Product2/2
  Sum2/1 -> Vector Concatenate1/1
  Gain/1 -> Vector Concatenate/2
  Sum3/1 -> Gain1/1
  Product4/1 -> Sum4/2
  Constant2/1 -> Vector Concatenate/1
  Sum5/1 -> Vector Concatenate2/2
  Vector Concatenate/1 -> Matrix Concatenate/1
  Product/1 -> Sum/2
  Sum1/1 -> Vector Concatenate/3
  Constant14/1 -> Sum5/1
  Gain1/1 -> Vector Concatenate1/3
  Gain2/1 -> Vector Concatenate2/1
  Constant5/1 -> Sum1/1
  Sum4/1 -> Gain2/1
  Matrix Concatenate/1 -> A_epsilon/1
  Random Number1/1 -> Product1/1
  Random Number2/1 -> Product2/1
  Random Number3/1 -> Product3/1
  Random Number4/1 -> Product4/1
  Random Number5/1 -> Product5/1

== system Model/Subsystem1/w_hat ==
  w_x : Inport
  w_y : Inport  Port=2
  w_z : Inport  Port=3
  Matrix Concatenate : Concatenate  NumInputs=3  Mode=Multidimensional array  ConcatenateDimension=2
  Scope : Scope  NumInputPorts=3
  Subsystem : Subsystem
  Subsystem1 : Subsystem
  Subsystem2 : Subsystem
  w_hat : Outport
  wires:
  w_y/1 -> Subsystem1/2(w_y), Subsystem/2(w_y), Subsystem2/2(w_y), Scope/2
  w_z/1 -> Subsystem2/3(w_z), Subsystem/3(w_z), Subsystem1/3(w_z), Scope/3
  w_x/1 -> Subsystem2/1(w_x), Subsystem/1(w_x), Subsystem1/1(w_x), Scope/1
  Subsystem2/1(Out1) -> Matrix Concatenate/3
  Subsystem1/1(Out1) -> Matrix Concatenate/2
  Subsystem/1(Out1) -> Matrix Concatenate/1
  Matrix Concatenate/1 -> w_hat/1

== system Model/A313/A(:,1)/Subsystem ==
  phi : Inport
  theta : Inport  Port=2
  psi : Inport  Port=3
  Cos18 : Trigonometry  Operator=cos
  Cos19 : Trigonometry  Operator=cos
  Cos20 : Trigonometry  Operator=cos
  Dot Product23 : DotProduct  InputSameDT=on  OutDataTypeStr=Inherit: Inherit via internal rule
  Product : Product  Inputs=3
  Sin16 : Trigonometry
  Sin17 : Trigonometry
  Sum8 : Sum  Inputs=+-
  A(1,1) : Outport
  wires:
  psi/1 -> Sin16/1, Cos18/1
  Dot Product23/1 -> Sum8/1
  Sin16/1 -> Product/1
  Cos18/1 -> Dot Product23/2
  Sin17/1 -> Product/2
  Cos19/1 -> Dot Product23/1
  Product/1 -> Sum8/2
  Sum8/1 -> A(1,1)/1  "A(1,1)"
  Cos20/1 -> Product/3
  phi/1 -> Cos19/1, Sin17/1
  theta/1 -> Cos20/1

== system Model/A313/A(:,1)/Subsystem1 ==
  phi : Inport
  theta : Inport  Port=2
  psi : Inport  Port=3
  Cos : Trigonometry  Operator=cos
  Cos1 : Trigonometry  Operator=cos
  Cos2 : Trigonometry  Operator=cos
  Dot Product : DotProduct  InputSameDT=on  OutDataTypeStr=Inherit: Inherit via internal rule
  Gain : Gain  Gain=-1
  Product : Product  Inputs=3
  Sin : Trigonometry
  Sin1 : Trigonometry
  Sum : Sum  Inputs=+-
  A(2,1) : Outport
  wires:
  psi/1 -> Cos1/1, Gain/1
  phi/1 -> Cos/1, Sin1/1
  Gain/1 -> Sin/1
  Cos/1 -> Dot Product/1
  Sin/1 -> Dot Product/2
  theta/1 -> Cos2/1
  Cos1/1 -> Product/1
  Sin1/1 -> Product/2
  Cos2/1 -> Product/3
  Dot Product/1 -> Sum/1
  Product/1 -> Sum/2
  Sum/1 -> A(2,1)/1  "A(2,1)"

== system Model/A313/A(:,1)/Subsystem2 ==
  phi : Inport
  theta : Inport  Port=2
  Dot Product : DotProduct  InputSameDT=on  OutDataTypeStr=Inherit: Inherit via internal rule
  Sin : Trigonometry
  Sin1 : Trigonometry
  A(3,1) : Outport
  wires:
  phi/1 -> Sin/1
  theta/1 -> Sin1/1
  Sin/1 -> Dot Product/1
  Sin1/1 -> Dot Product/2
  Dot Product/1 -> A(3,1)/1

== system Model/A313/A(:,2)/Subsystem3 ==
  phi : Inport
  theta : Inport  Port=2
  psi : Inport  Port=3
  Cos18 : Trigonometry  Operator=cos
  Cos19 : Trigonometry  Operator=cos
  Cos20 : Trigonometry  Operator=cos
  Dot Product : DotProduct  InputSameDT=on  OutDataTypeStr=Inherit: Inherit via internal rule
  Product : Product  Inputs=3
  Sin16 : Trigonometry
  Sin17 : Trigonometry
  Sum : Sum  Inputs=|++
  A(1,2) : Outport
  wires:
  Cos18/1 -> Dot Product/2
  phi/1 -> Cos19/1, Sin16/1
  psi/1 -> Cos18/1, Sin17/1
  Sin16/1 -> Dot Product/1
  theta/1 -> Cos20/1
  Sin17/1 -> Product/1
  Cos19/1 -> Product/2
  Cos20/1 -> Product/3
  Dot Product/1 -> Sum/1
  Product/1 -> Sum/2
  Sum/1 -> A(1,2)/1

== system Model/A313/A(:,2)/Subsystem4 ==
  phi : Inport
  theta : Inport  Port=2
  psi : Inport  Port=3
  Cos : Trigonometry  Operator=cos
  Cos1 : Trigonometry  Operator=cos
  Cos2 : Trigonometry  Operator=cos
  Dot Product : DotProduct  InputSameDT=on  OutDataTypeStr=Inherit: Inherit via internal rule
  Product : Product  Inputs=3
  Sin : Trigonometry
  Sin1 : Trigonometry
  Sum : Sum  Inputs=-+
  A(2,2) : Outport
  wires:
  phi/1 -> Sin1/1, Cos/1
  psi/1 -> Cos1/1, Sin/1
  Sin1/1 -> Dot Product/1
  Sin/1 -> Dot Product/2
  theta/1 -> Cos2/1
  Cos2/1 -> Product/2
  Cos/1 -> Product/1
  Cos1/1 -> Product/3
  Dot Product/1 -> Sum/1
  Product/1 -> Sum/2
  Sum/1 -> A(2,2)/1

== system Model/A313/A(:,2)/Subsystem5 ==
  phi : Inport
  theta : Inport  Port=2
  Cos : Trigonometry  Operator=cos
  Dot Product : DotProduct  InputSameDT=on  OutDataTypeStr=Inherit: Inherit via internal rule
  Gain : Gain  Gain=-1
  Sin : Trigonometry
  A(3,2) : Outport
  wires:
  phi/1 -> Cos/1
  theta/1 -> Sin/1
  Cos/1 -> Dot Product/1
  Sin/1 -> Dot Product/2
  Dot Product/1 -> Gain/1
  Gain/1 -> A(3,2)/1

== system Model/A313/A(:,3)/Subsystem6 ==
  theta : Inport
  psi : Inport  Port=2
  Dot Product : DotProduct  InputSameDT=on  OutDataTypeStr=Inherit: Inherit via internal rule
  Sin : Trigonometry
  Sin1 : Trigonometry
  A(1,3) : Outport
  wires:
  psi/1 -> Sin/1
  theta/1 -> Sin1/1
  Dot Product/1 -> A(1,3)/1
  Sin1/1 -> Dot Product/1
  Sin/1 -> Dot Product/2

== system Model/A313/A(:,3)/Subsystem7 ==
  theta : Inport
  psi : Inport  Port=2
  Dot Product : DotProduct  InputSameDT=on  OutDataTypeStr=Inherit: Inherit via internal rule
  Sin : Trigonometry  Operator=cos
  Sin1 : Trigonometry
  A(2,3) : Outport
  wires:
  psi/1 -> Sin/1
  theta/1 -> Sin1/1
  Dot Product/1 -> A(2,3)/1
  Sin1/1 -> Dot Product/1
  Sin/1 -> Dot Product/2

== system Model/A313/A(:,3)/Subsystem8 ==
  theta : Inport
  Cos18 : Trigonometry  Operator=cos
  A(3,3) : Outport
  wires:
  theta/1 -> Cos18/1
  Cos18/1 -> A(3,3)/1

== system Model/A_L//N/first column of A_L//N/argument of periodic functions ==
  Clock : Clock
  Constant : Constant  Value=n
  Dot Product : DotProduct  InputSameDT=on  OutDataTypeStr=Inherit: Inherit via internal rule
  n*t : Outport
  wires:
  Clock/1 -> Dot Product/1
  Dot Product/1 -> n*t/1
  Constant/1 -> Dot Product/2

== system Model/A_L//N/first column of A_L//N/argument of periodic functions1 ==
  Clock : Clock
  Constant : Constant  Value=n
  Dot Product : DotProduct  InputSameDT=on  OutDataTypeStr=Inherit: Inherit via internal rule
  n*t : Outport
  wires:
  Clock/1 -> Dot Product/1
  Dot Product/1 -> n*t/1
  Constant/1 -> Dot Product/2

== system Model/A_L//N/second column of A_L//N/argument of periodic functions ==
  Clock : Clock
  Constant : Constant  Value=n
  Dot Product : DotProduct  InputSameDT=on  OutDataTypeStr=Inherit: Inherit via internal rule
  n*t : Outport
  wires:
  Clock/1 -> Dot Product/1
  Dot Product/1 -> n*t/1
  Constant/1 -> Dot Product/2

== system Model/A_L//N/second column of A_L//N/argument of periodic functions1 ==
  Clock : Clock
  Constant : Constant  Value=n
  Dot Product : DotProduct  InputSameDT=on  OutDataTypeStr=Inherit: Inherit via internal rule
  n*t : Outport
  wires:
  Clock/1 -> Dot Product/1
  Dot Product/1 -> n*t/1
  Constant/1 -> Dot Product/2
